simulink model "IPMSMOuterLoopControl"  (R2025a)
settings: Solver=VariableStepAuto  StartTime=0.0  StopTime=3  FixedStep=Ts  RelTol=1e-3  EnableMultiTasking=on
PreLoadFcn:
  | IPMSMOuterLoopControlData;
values from neighbouring files (symbols this model uses):
  p = 8    [IPMSMOuterLoopControlData.m]
  Ts = 1e-4    (= 0.0001)    [IPMSMOuterLoopControlData.m]
  Tso = 1e-3    (= 0.001)    [IPMSMOuterLoopControlData.m]
libraries: fl_lib x8, nesl_utility x7, ee_lib x3, eeTransforms x1, eePmsmCurrentReferenceGen x1, eeVelocityController x1, SignalEditorBlockLib x1
CloseFcn:
  | try,close(h1_IPMSMOuterLoopControl),end
  | clear h1_IPMSMOuterLoopControl
  | 
  | clear simlog_IPMSMOuterLoopControl
  | clear logsout_IPMSMOuterLoopControl
  | 
  | clear dend_omega ID_MAP IQ_MAP
  | clear Jm Ki_omega Kp_omega L0 Ld Lq numd_omega p Pmax
  | clear psim RPM_VECT Rs Tmax tout TQ_VECT Ts Tso VDC_VECT Vnom
Description:
  | IPMSM Outer Loop Controller Evaluation
settings Model: Creator=The MathWorks, Inc.  LastModifiedBy=ransr
settings SolverCC: AlgebraicLoopSolver=TrustRegion  AutoInsertRateTranBlk=on  MaxZcPerStep=1.0
settings DataIOCC: MaxDataPoints=210000  ReturnWorkspaceOutputs=off  SignalLoggingName=logsout_IPMSMOuterLoopControl
settings OptimizationCC: ReuseModelBlockBuffer=off  LifeSpan=inf
settings DebuggingCC: UnconnectedInputMsg=warning  UnconnectedOutputMsg=warning  UnconnectedLineMsg=warning  SFUnexpectedBacktrackingDiag=warning  SFNoUnconditionalDefaultTransitionDiag=warning  SFExecutionAtInitializationDiag=none  ArithmeticOperatorsInVariantConditions=warning
settings ModelReferenceCC: EnableRefExpFcnMdlSchedulingChecks=on
settings SFSimCC: SimUseLocalCustomCode=off  CustomCodeUndefinedFunction=UseInterfaceOnly
settings RTWCC: RTWUseLocalCustomCode=off  GPUComputeCapability=3.5  DLArmComputeVersion=19.05
settings CodeAppCC: StateflowObjectComments=on
settings GRTTargetCC: TargetLangStandard=C89/C90 (ANSI)
settings ConfigComp: CovMetricSettings=dw  CovSaveCumulativeToWorkspaceVar=on  CovSaveSingleToWorkspaceVar=on  CovExternalEMLEnable=off
settings SimscapeCC: SimscapeNormalizeSystem=off  SimscapeLogType=all  SimscapeLogSimulationStatistics=on  SimscapeLogName=simlog_IPMSMOuterLoopControl  SimscapeLogDataHistory=210000.0

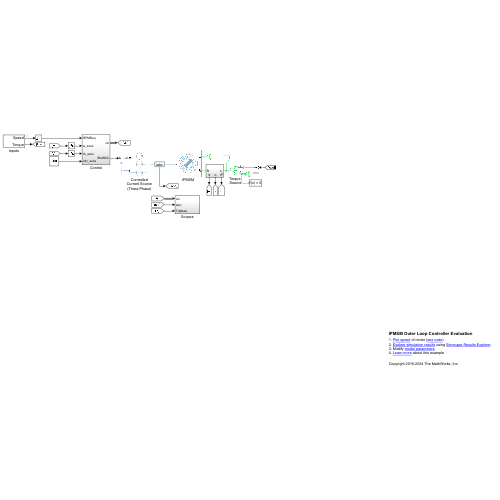
[thumbnail: Simulink's stored preview of the top-level diagram]
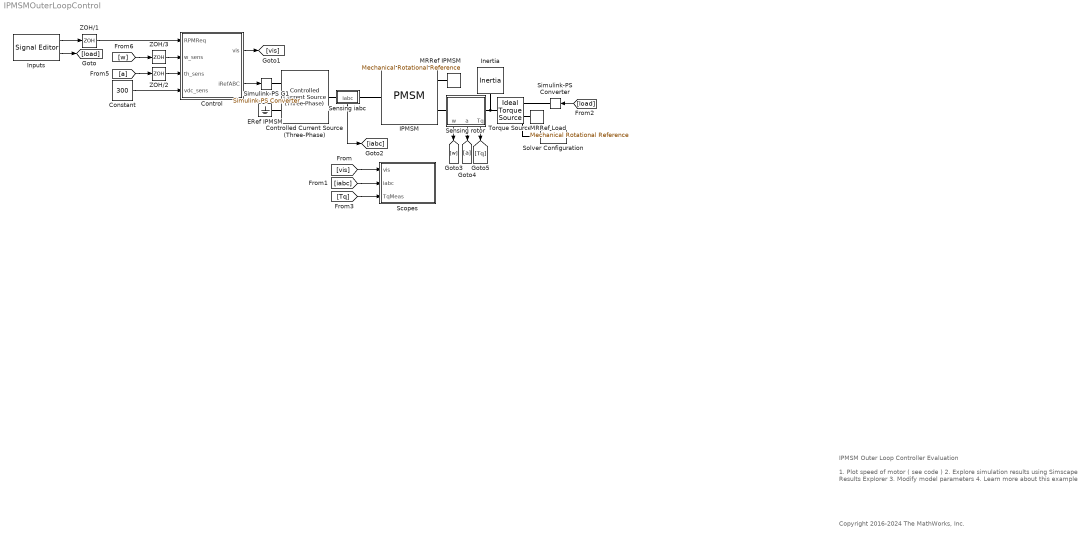
== system IPMSMOuterLoopControl ==
  note: IPMSM Outer Loop Controller Evaluation
  note: 1. Plot speed of motor ( see code )
      | 2. Explore simulation results using Simscape Results Explorer
      | 3. Modify model parameters
      | 4. Learn more about this example
  note: Copyright 2016-2024 The MathWorks, Inc.
  Constant : Constant  Value=300
  Control : Subsystem
  Controlled Current Source (Three-Phase) : ee_lib/Sources/Controlled Current Source (Three-Phase)  input_option=ee.enum.inputType.instantaneous  FRated=60 Hz
      settings: InternalSimscapePortConfiguration="{\"Bottom\":[],\"Left\":[{\"id\":\"S\",\"label\":\"S\",\"type\":\"input\"},{\"id\":\"n\",\"label\":\"n\",\"type\":\"foundation.electrical.electrical\"}],\"Right\":[{\"id\":\"N\",\"label\":\"~\",\"type\":\"foundation.electrical.three_phase\"}],\"Top\":[]}"
  ERef IPMSM : fl_lib/Electrical/Electrical Elements/Electrical Reference
  IPMSM : ee_lib/Electromechanical/Permanent Magnet/PMSM  port_option=ee.enum.threePhasePort.composite  winding_type=ee.enum.statorconnection.wye  machine_param=ee.enum.pmsm.parameterization.constant  nPolePairs=p  pmflux_param=ee.enum.pmflux.fluxlinkage  pm_flux_linkage=psim Wb  torque_constant=0.18 N*m/A  back_emf_constant=0.18 V/(rad/s)  stator_param=1  Ld=Ld H  Lq=Lq H  idVec=[-200, 0, 200] A  iqVec=[-200, 0, 200] A  LdMatrix=0.0002 * ones(3, 3) H  LqMatrix=0.0002 * ones(3, 3) H  PmMatrix=0.1 * ones(3, 3) Wb  ktMatrix=0.18 * ones(3, 3) N*m/A  keMatrix=0.18 * ones(3, 3) V/(rad/s)  L0=L0 H  Ls=0.0002 H  Lm=0.00002 H  Ms=0.00002 H  Rs=Rs Ohm  zero_sequence=ee.enum.park.zerosequence.exclude  axes_param=ee.enum.rotorangle.qaxis  loss_param=ee.enum.ironloss.empirical  losses_oc=[0, 0, 0] W  losses_sc=[0, 0, 0] W  f_losses=60 Hz  Isc_losses=95 A  J=0 kg*m^2  lam=0 N*m/(rad/s)  i_d_specify=off  i_d_priority=None  i_d=0 A  i_d_nominal_specify=off  i_d_nominal_value=1  i_d_nominal_unit=A  i_q_specify=off  i_q_priority=None  i_q=0 A  i_q_nominal_specify=off  i_q_nominal_value=1  i_q_nominal_unit=A  torque_specify=off  torque_priority=None  torque=0 N*m  torque_nominal_specify=off  torque_nominal_value=1  torque_nominal_unit=N*m  angular_velocity_specify=on  angular_velocity_priority=None  angular_velocity=0 rpm  angular_velocity_nominal_specify=off  angular_velocity_nominal_value=1  angular_velocity_nominal_unit=rpm  angular_position_specify=on  angular_position_priority=None  angular_position=0 rad  angular_position_nominal_specify=off  angular_position_nominal_value=1  angular_position_nominal_unit=deg  alpha=3.93e-3 1/K  alpha_flux=-0.001 1/K  Tmeas=298.15 K  stator_thermal_mass=100 J/K  rotor_thermal_mass=200 J/K  Rm_percent_rotor=90  Rd_percent_rotor=30  temperatureA_specify=off  temperatureA_priority=High  temperatureA=25 degC  temperatureA_nominal_specify=off  temperatureA_nominal_value=1  temperatureA_nominal_unit=degC  temperatureB_specify=off  temperatureB_priority=High  temperatureB=25 degC  temperatureB_nominal_specify=off  temperatureB_nominal_value=1  temperatureB_nominal_unit=degC  temperatureC_specify=off  temperatureC_priority=High  temperatureC=25 degC  temperatureC_nominal_specify=off  temperatureC_nominal_value=1  temperatureC_nominal_unit=degC  temperatureR_specify=off  temperatureR_priority=High  temperatureR=25 degC  temperatureR_nominal_specify=off  temperatureR_nominal_value=1  temperatureR_nominal_unit=degC
      settings: InternalSimscapePortConfiguration="{\"Bottom\":[],\"Left\":[{\"id\":\"N\",\"label\":\"~\",\"type\":\"foundation.electrical.three_phase\"}],\"Right\":[{\"id\":\"R\",\"label\":\"R\",\"type\":\"foundation.mechanical.rotational.rotational\"},{\"id\":\"C\",\"label\":\"C\",\"type\":\"foundation.mechanical.rotational.rotational\"}],\"Top\":[]}"
  Inertia : fl_lib/Mechanical/Rotational Elements/Inertia  inertia=Jm kg*m^2  num_ports=foundation.enum.numPorts2.one  w_specify=on  w_priority=None  w=0 rad/s  w_nominal_specify=off  w_nominal_value=1  w_nominal_unit=rad/s  t_specify=off  t_priority=High  t=0 N*m  t_nominal_specify=off  t_nominal_value=1  t_nominal_unit=N*m
  Inputs : SignalEditorBlockLib/Signal Editor  FileName=inputs.mat  ActiveScenario=Test_1  ActiveSignal=Torque  IsBus=off  OutputBusObjectStr=Bus: BusObject  SampleTime=49.28727583451705  OutputAfterFinalValue=Extrapolation  Unit=inherit  PreserveSignalName=on  ApplySigPropsToAllScenarios=on  ApplySigPropsToAllSignals=off  SignalPropertySource=Dialog parameters
  MRRef IPMSM : fl_lib/Mechanical/Rotational Elements/Mechanical Rotational Reference
  MRRef Load : fl_lib/Mechanical/Rotational Elements/Mechanical Rotational Reference
  Scopes : Subsystem
  Sensing rotor : Subsystem
      settings: PortSchema="{\"entries\":[{\"content\":{\"sides\":[{\"content\":{\"connectorIds\":[\"LConn1\"]},\"type\":\"ConnectorPlacement.EquallySpacedRectSide\",\"uuid\":\"46201c8d-77b1-447d-9042-ac8be5c0bd79\"},{\"content\":{\"connectorIds\":[\"RConn1\"],\"side\":\"RIGHT\"},\"type\":\"ConnectorPlacement.EquallySpacedRectSide\",\"uuid\":\"936c7aef-5ef9-4b0b-b575-5e9b10060a4e\"},{\"content\":{\"connectorIds\":[],\"side\":\"TOP\"},\"type\":\"ConnectorPlacement.EquallySpacedRectSide\",\"uuid\":\"45660790-80d7-41be-a100-9c6aa98be58d\"},{\"content\":{\"connectorIds\":[\"Out1\",\"Out2\",\"Out3\"],\"side\":\"BOTTOM\"},\"type\":\"ConnectorPlacement.EquallySpacedRectSide\",\"uuid\":\"46e277bc-d0fb-476a-ab18-81dc7f8b176e\"}]},\"type\":\"ConnectorPlacement.EquallySpacedConnector\",\"uuid\":\"bf9a60fc-c3c6-4698-a696-692df8c6cda0\"}],\"packageUris\":[\"http://schema.mathworks.com/mf0/Connector/R2020b\"],\"version\":\"1.0\"}"
  Sensing iabc : Subsystem
      settings: PortSchema="{\"entries\":[{\"content\":{\"sides\":[{\"content\":{\"connectorIds\":[\"LConn1\"]},\"type\":\"ConnectorPlacement.EquallySpacedRectSide\",\"uuid\":\"d65c841b-b32b-49bd-9628-387529d43346\"},{\"content\":{\"connectorIds\":[\"RConn1\"],\"side\":\"RIGHT\"},\"type\":\"ConnectorPlacement.EquallySpacedRectSide\",\"uuid\":\"6cf26a03-8bd2-4d9d-a8e8-cf9c158ad2d5\"},{\"content\":{\"connectorIds\":[],\"side\":\"TOP\"},\"type\":\"ConnectorPlacement.EquallySpacedRectSide\",\"uuid\":\"233452df-4576-4294-a118-5720dbcd2b4b\"},{\"content\":{\"connectorIds\":[\"Out1\"],\"side\":\"BOTTOM\"},\"type\":\"ConnectorPlacement.EquallySpacedRectSide\",\"uuid\":\"626b4b83-21f3-4703-b002-a76396a072ce\"}]},\"type\":\"ConnectorPlacement.EquallySpacedConnector\",\"uuid\":\"c5331da1-3503-4f87-b285-4d520d369061\"}],\"packageUris\":[\"http://schema.mathworks.com/mf0/Connector/R2020b\"],\"version\":\"1.0\"}"
      mask Display: disp('iabc')
  Simulink-PS Converter : nesl_utility/Simulink-PS Converter  PhysicalDomain=network_engine_domain  SubClassName=ps_input  LeftPortType=input  RightPortType=output  PseudoPeriodic=off  Frequencies=[]  NoiseDistribution=none  NoiseParameters=[]  Unit=N*m  AffineConversion=off  FilteringAndDerivatives=zero  SimscapeFilterOrder=1  InputFilterTimeConstant=0.001  UdotUserProvided=1
  Simulink-PS G1 : nesl_utility/Simulink-PS Converter  PhysicalDomain=network_engine_domain  SubClassName=ps_input  LeftPortType=input  RightPortType=output  PseudoPeriodic=off  Frequencies=[]  NoiseDistribution=none  NoiseParameters=[]  Unit=A  AffineConversion=off  FilteringAndDerivatives=zero  SimscapeFilterOrder=1  InputFilterTimeConstant=1e-6  UdotUserProvided=1
  Solver Configuration : nesl_utility/Solver Configuration  PhysicalDomain=network_engine_domain  SubClassName=solver  LeftPortType=input  RightPortType=generic  Tones=[]  Harmonics=[]  SimulateNoise=off  Profile=off  UseLocalSampling=off  EnableSwitchedLinearOptims=on  FrequencyDomain=off  UseCCode=off  RelTol=0.001  AbsTol=1e-06  MinStep=1e-09  ToWorkspace=off  RevertToSquareIcSolve=off  NumHomotopyIterations=100  PhasorMode=off  PhasorModeNumHarmonics=1  ConsistencySolver=NEWTON_FTOL  IndexReductionMethod=DerivativeReplacement  DoDC=off  ResidualTolerance=1e-9  ConsistencyTolSource=GLOBAL  ConsistencyAbsTol=0.001  ConsistencyRelTol=0.001  ConsistencyTolFactor=0.001  UseLocalSolver=on  LocalSolverChoice=NE_BACKWARD_EULER_ADVANCER  ResolveIndetEquations=on  FunctionEvalNumThread=1  LocalSolverSampleTime=Ts  DoFixedCost=on  MaxNonlinIter=3  MaxModeIter=2  ComputeImpulses=off  ImpulseIterations=2  LinearAlgebra=auto  LinearAlgebraNumThread=0  EquationFormulation=NE_TIME_EF  DelaysMemoryBudget=1024  AutomaticFiltering=on  FilteringTimeConstant=0.001  PartitionStorageMethod=AS_NEEDED  PartitionMemoryBudget=1024  PartitionMethod=FAST  MultibodyUseLocalSolver=off  MultibodyLocalSolverChoice=ODE1  MultibodyLocalSolverSampleTime=0.001
  Torque Source : fl_lib/Mechanical/Mechanical Sources/Ideal Torque Source
  ZOH/1 : ZeroOrderHold  SampleTime=Tso
  ZOH/2 : ZeroOrderHold  SampleTime=Ts
  ZOH/3 : ZeroOrderHold  SampleTime=Tso
  wires:
  [load] -> Simulink-PS Converter/1
  Inputs/1 -> ZOH/1/1
  Constant/1 -> Control/4(vdc_sens)
  [w] -> ZOH/3/1
  [a] -> ZOH/2/1
  Inputs/2 -> [load]
  ZOH/1/1 -> Control/1(RPMReq)
  ZOH/3/1 -> Control/2(w_sens)
  ZOH/2/1 -> Control/3(th_sens)
  Control/2(iRefABC) -> Simulink-PS G1/1
  Control/1(vis) -> [vis]
  [vis] -> Scopes/1(vis)
  Sensing iabc/1(iabc) -> [iabc]
  [iabc] -> Scopes/2(iabc)
  Sensing rotor/1(w) -> [w]
  Sensing rotor/2(a) -> [a]
  Sensing rotor/3(Tq) -> [Tq]
  [Tq] -> Scopes/3(TqMeas)
  connections:
  Torque Source/LConn1 -- Inertia/LConn1 -- Sensing rotor/RConn1
  Torque Source/RConn1 -- Simulink-PS Converter/RConn1
  Torque Source/RConn2 -- Solver Configuration/RConn1 -- MRRef Load/LConn1
  Sensing iabc/RConn1 -- IPMSM/LConn1
  IPMSM/RConn2 -- MRRef IPMSM/LConn1
  IPMSM/RConn1 -- Sensing rotor/LConn1
  Simulink-PS G1/RConn1 -- Controlled Current Source (Three-Phase)/LConn1
  Controlled Current Source (Three-Phase)/RConn1 -- Sensing iabc/LConn1
  ERef IPMSM/LConn1 -- Controlled Current Source (Three-Phase)/LConn2

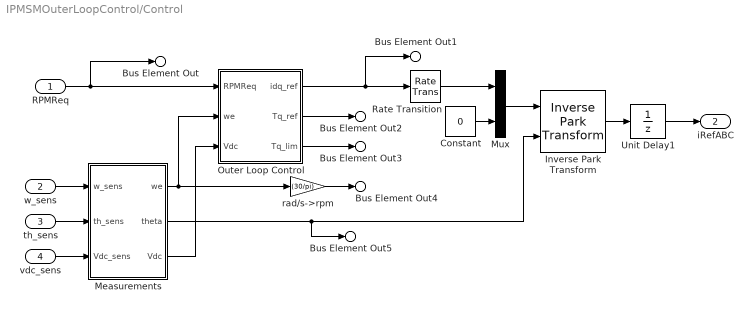
== system IPMSMOuterLoopControl/Control ==
  RPMReq : Inport
  w_sens : Inport  Port=2
  th_sens : Inport  Port=3
  vdc_sens : Inport  Port=4
  Constant : Constant  Value=0  SampleTime=Ts
  Inverse Park Transform : eeTransforms/Inverse Park Transform  AxisAlignment=Q-axis  PowerInvariant=off
  Measurements : Subsystem
  Mux : Mux  Inputs=2
  Outer Loop Control : Subsystem
  Rate Transition : RateTransition  OutPortSampleTime=Ts
  Unit Delay1 : UnitDelay  SampleTime=Ts  HasFrameUpgradeWarning=on
  rad/s->rpm : Gain  Gain=(30/pi)
  Bus Element Out : Outport  PortName=vis  Element=spdRef
  Bus Element Out1 : Outport  PortName=vis  Element=idqRef
  Bus Element Out2 : Outport  PortName=vis  Element=TqRef
  Bus Element Out3 : Outport  PortName=vis  Element=TqLim
  Bus Element Out4 : Outport  PortName=vis  Element=spd
  Bus Element Out5 : Outport  PortName=vis  Element=theta
  iRefABC : Outport  Port=2  VectorParamsAs1DForOutWhenUnconnected=off
  wires:
  Outer Loop Control/1(idq_ref) -> Rate Transition/1, Bus Element Out1/1
  w_sens/1 -> Measurements/1(w_sens)
  th_sens/1 -> Measurements/2(th_sens)
  vdc_sens/1 -> Measurements/3(Vdc_sens)
  RPMReq/1 -> Bus Element Out/1, Outer Loop Control/1(RPMReq)
  Measurements/3(Vdc) -> Outer Loop Control/3(Vdc)
  Outer Loop Control/2(Tq_ref) -> Bus Element Out2/1
  Measurements/1(we) -> rad/s->rpm/1, Outer Loop Control/2(we)
  rad/s->rpm/1 -> Bus Element Out4/1
  Outer Loop Control/3(Tq_lim) -> Bus Element Out3/1
  Measurements/2(theta) -> Bus Element Out5/1, Inverse Park Transform/2
  Rate Transition/1 -> Mux/1
  Inverse Park Transform/1 -> Unit Delay1/1
  Constant/1 -> Mux/2
  Mux/1 -> Inverse Park Transform/1
  Unit Delay1/1 -> iRefABC/1

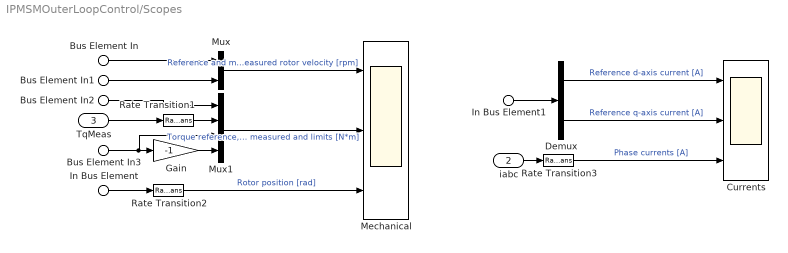
== system IPMSMOuterLoopControl/Scopes ==
  Bus Element In : Inport  PortName=vis  Element=spdRef
  Bus Element In1 : Inport  PortName=vis  Element=spd
  Bus Element In2 : Inport  PortName=vis  Element=TqRef
  Bus Element In3 : Inport  PortName=vis  Element=TqLim
  In Bus Element : Inport  PortName=vis  Element=theta
  In Bus Element1 : Inport  PortName=vis  Element=idqRef
  iabc : Inport  Port=2
  TqMeas : Inport  Port=3
  Currents : Scope  NumInputPorts=3
      settings: ActiveDisplayYMinimum=-303.05966313651174  ActiveDisplayYMaximum=237.72746096569756  DataLoggingSaveFormat=Array
  Demux : Demux  Outputs=2
  Gain : Gain  Gain=-1
  Mechanical : Scope  NumInputPorts=3
      settings: ActiveDisplayYMinimum=-824.87134285736943  ActiveDisplayYMaximum=7272.1659214876536  DataLoggingVariableName=ScopeData5  DataLoggingSaveFormat=Array
  Mux : Mux  Inputs=2
  Mux1 : Mux
  Rate Transition1 : RateTransition  OutPortSampleTime=Tso
  Rate Transition2 : RateTransition  OutPortSampleTime=Tso
  Rate Transition3 : RateTransition  OutPortSampleTime=Tso
  wires:
  Bus Element In1/1 -> Mux/2
  Gain/1 -> Mux1/4
  Bus Element In2/1 -> Mux1/1
  iabc/1 -> Rate Transition3/1
  Bus Element In/1 -> Mux/1
  TqMeas/1 -> Rate Transition1/1
  Demux/1 -> Currents/1  "Reference d-axis current [A]"
  Bus Element In3/1 -> Mux1/3, Gain/1
  Mux1/1 -> Mechanical/2  "Torque reference, measured and limits [N*m]"
  In Bus Element/1 -> Rate Transition2/1
  Rate Transition1/1 -> Mux1/2
  Mux/1 -> Mechanical/1  "Reference and measured rotor velocity [rpm]"
  In Bus Element1/1 -> Demux/1
  Demux/2 -> Currents/2  "Reference q-axis current [A]"
  Rate Transition2/1 -> Mechanical/3  "Rotor position [rad]"
  Rate Transition3/1 -> Currents/3  "Phase currents [A]"

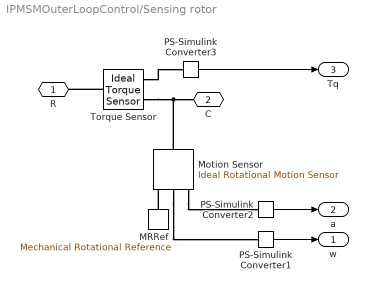
== system IPMSMOuterLoopControl/Sensing rotor ==
  MRRef : fl_lib/Mechanical/Rotational Elements/Mechanical Rotational Reference
  Motion Sensor : fl_lib/Mechanical/Mechanical Sensors/Ideal Rotational Motion Sensor  reference=foundation.enum.MeasurementReference.difference  acceleration_port=false  velocity_port=true  position_port=true  wrap_angle=simscape.enum.onoff.off  offset=0 deg
  PS-Simulink Converter1 : nesl_utility/PS-Simulink Converter  PhysicalDomain=network_engine_domain  SubClassName=ps_output  LeftPortType=input  RightPortType=output  PseudoPeriodic=off  Frequencies=[]  VectorFormat=1-D array  Unit=rad/s  AffineConversion=off
  PS-Simulink Converter2 : nesl_utility/PS-Simulink Converter  PhysicalDomain=network_engine_domain  SubClassName=ps_output  LeftPortType=input  RightPortType=output  PseudoPeriodic=off  Frequencies=[]  VectorFormat=1-D array  Unit=rad  AffineConversion=off
  PS-Simulink Converter3 : nesl_utility/PS-Simulink Converter  PhysicalDomain=network_engine_domain  SubClassName=ps_output  LeftPortType=input  RightPortType=output  PseudoPeriodic=off  Frequencies=[]  VectorFormat=1-D array  Unit=N*m  AffineConversion=off
  Torque Sensor : fl_lib/Mechanical/Mechanical Sensors/Ideal Torque Sensor
  R : PMIOPort  Side=Left
  C : PMIOPort  Port=2  Side=Right
  w : Outport
  a : Outport  Port=2
  Tq : Outport  Port=3
  wires:
  PS-Simulink Converter3/1 -> Tq/1
  PS-Simulink Converter1/1 -> w/1
  PS-Simulink Converter2/1 -> a/1
  connections:
  Torque Sensor/RConn1 -- Motion Sensor/LConn1 -- C/RConn1
  Torque Sensor/RConn2 -- PS-Simulink Converter3/LConn1
  Torque Sensor/LConn1 -- R/RConn1
  MRRef/LConn1 -- Motion Sensor/RConn1
  Motion Sensor/RConn3 -- PS-Simulink Converter2/LConn1
  Motion Sensor/RConn2 -- PS-Simulink Converter1/LConn1

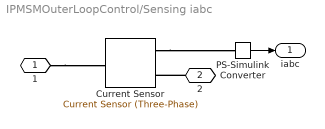
== system IPMSMOuterLoopControl/Sensing iabc ==
  Current Sensor : ee_lib/Sensors & Transducers/Current Sensor (Three-Phase)
  PS-Simulink Converter : nesl_utility/PS-Simulink Converter  PhysicalDomain=network_engine_domain  SubClassName=ps_output  LeftPortType=input  RightPortType=output  PseudoPeriodic=off  Frequencies=[]  VectorFormat=1-D array  Unit=A  AffineConversion=off
  1 : PMIOPort  Side=Left
  2 : PMIOPort  Port=2  Side=Right
  iabc : Outport
  wires:
  PS-Simulink Converter/1 -> iabc/1
  connections:
  1/RConn1 -- Current Sensor/LConn1
  2/RConn1 -- Current Sensor/RConn2
  Current Sensor/RConn1 -- PS-Simulink Converter/LConn1

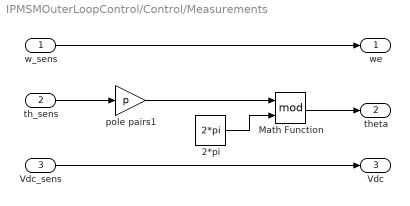
== system IPMSMOuterLoopControl/Control/Measurements ==
  w_sens : Inport
  th_sens : Inport  Port=2
  Vdc_sens : Inport  Port=3
  2*pi : Constant  Value=2*pi  SampleTime=-1
  Math Function : Math  Operator=mod  SignedPower=on
  "pole pairs1 " : Gain  Gain=p
  we : Outport  VectorParamsAs1DForOutWhenUnconnected=off
  theta : Outport  Port=2  VectorParamsAs1DForOutWhenUnconnected=off
  Vdc : Outport  Port=3  VectorParamsAs1DForOutWhenUnconnected=off
  wires:
  w_sens/1 -> we/1
  th_sens/1 -> "pole pairs1 "/1
  "pole pairs1 "/1 -> Math Function/1
  2*pi/1 -> Math Function/2
  Math Function/1 -> theta/1
  Vdc_sens/1 -> Vdc/1

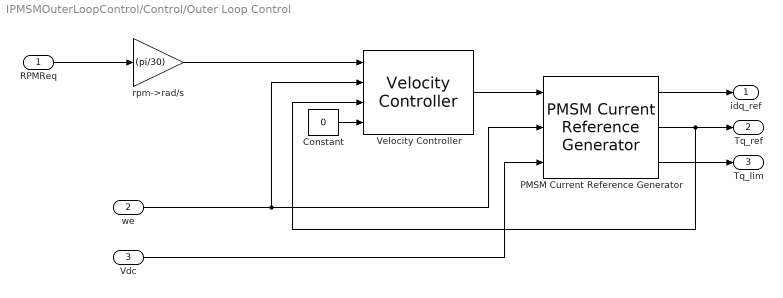
== system IPMSMOuterLoopControl/Control/Outer Loop Control ==
  RPMReq : Inport
  we : Inport  Port=2
  Vdc : Inport  Port=3
  Constant : Constant  Value=0  SampleTime=-1
  PMSM Current Reference Generator : eePmsmCurrentReferenceGen/PMSM Current Reference Generator  Vnom=Vnom  Pmax=Pmax  Tmax=Tmax  Ts=Tso  RefType=Lookup-table based  rpmVec=RPM_VECT  TqVec=TQ_VECT  VdcVec=VDC_VECT  PWMMode=SVM: space vector modulation  ModFactor=1  idMatrix=ID_MAP  iqMatrix=IQ_MAP  p=8  psim=0.04  Ld=0.00024  Lq=0.00029  Rs=0.01  RefExpEnable=0
  Velocity Controller : eeVelocityController/Velocity Controller  CtrlType=P-PI control  Kp_w=Kp_omega  Ki_w=Ki_omega  Kv_w=Kp_omega  Kaw_w=100  Ts=Tso  Tsd=Tso  ActZC=on
  rpm->rad/s : Gain  Gain=(pi/30)
  idq_ref : Outport  VectorParamsAs1DForOutWhenUnconnected=off
  Tq_ref : Outport  Port=2  VectorParamsAs1DForOutWhenUnconnected=off
  Tq_lim : Outport  Port=3  VectorParamsAs1DForOutWhenUnconnected=off
  wires:
  rpm->rad/s/1 -> Velocity Controller/1
  Velocity Controller/1 -> PMSM Current Reference Generator/1
  RPMReq/1 -> rpm->rad/s/1
  Vdc/1 -> PMSM Current Reference Generator/3
  PMSM Current Reference Generator/1 -> idq_ref/1
  PMSM Current Reference Generator/2 -> Tq_ref/1, Velocity Controller/3
  PMSM Current Reference Generator/3 -> Tq_lim/1
  we/1 -> PMSM Current Reference Generator/2, Velocity Controller/2
  Constant/1 -> Velocity Controller/4
